simulink model "Task5_Subtask_1"  (R2023b)
settings: Solver=FixedStepDiscrete  StartTime=0.0  StopTime=(16+168+1)*24  RelTol=1e-3
settings Model: LastModifiedBy=AMEY THAKUR

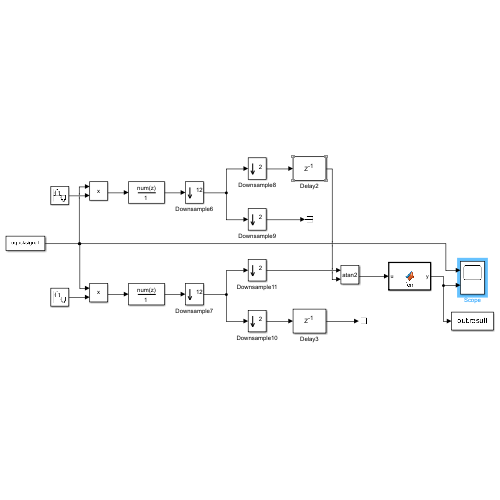
[thumbnail: Simulink's stored preview of the top-level diagram]
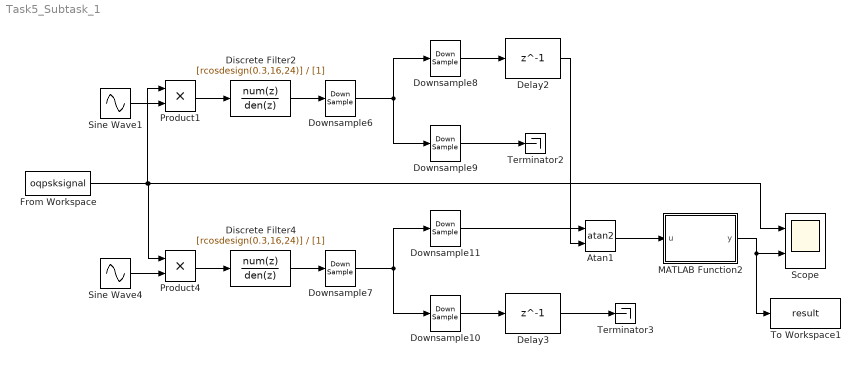
== system Task5_Subtask_1 ==
  Atan1 : Trigonometry  Operator=atan2
  Delay2 : Delay  DelayLength=1  UseCircularBuffer=on
  Delay3 : Delay  DelayLength=1  InitialCondition=0  UseCircularBuffer=on
  Discrete Filter2 : DiscreteFilter  Numerator=[rcosdesign(0.3,16,24)]  Denominator=[1]
  Discrete Filter4 : DiscreteFilter  Numerator=[rcosdesign(0.3,16,24)]  Denominator=[1]
  Downsample10 : DownSample  RateOptions=Allow multirate processing
  Downsample11 : DownSample  phase=1  RateOptions=Allow multirate processing
  Downsample6 : DownSample  N=12  RateOptions=Allow multirate processing
  Downsample7 : DownSample  N=12  RateOptions=Allow multirate processing
  Downsample8 : DownSample  RateOptions=Allow multirate processing
  Downsample9 : DownSample  phase=1  RateOptions=Allow multirate processing
  From Workspace : FromWorkspace  VariableName=oqpsksignal  SampleTime=1
  MATLAB Function2 : MATLAB Function  TreatAsAtomicUnit=on
  Product1 : Product
  Product4 : Product
  Scope : Scope  NumInputPorts=2
  Sine Wave1 : Sin  Amplitude=sqrt(2)  Frequency=2*pi*0.25  Phase=pi/2  SampleTime=1
  Sine Wave4 : Sin  Amplitude=-sqrt(2)  Frequency=2*pi*0.25  SampleTime=1
  Terminator2 : Terminator
  Terminator3 : Terminator
  To Workspace1 : ToWorkspace  VariableName=result  SampleTime=-1
      settings: Save2DSignal=2-D array (concatenate along first dimension)
  wires:
  Discrete Filter2/1 -> Downsample6/1
  Discrete Filter4/1 -> Downsample7/1
  Atan1/1 -> MATLAB Function2/1(u)
  Downsample10/1 -> Delay3/1
  Sine Wave4/1 -> Product4/2
  Product4/1 -> Discrete Filter4/1
  Downsample7/1 -> Downsample11/1, Downsample10/1
  Product1/1 -> Discrete Filter2/1
  Downsample9/1 -> Terminator2/1
  Downsample11/1 -> Atan1/1
  Delay3/1 -> Terminator3/1
  Sine Wave1/1 -> Product1/2
  MATLAB Function2/1(y) -> Scope/2, To Workspace1/1
  Downsample8/1 -> Delay2/1
  Downsample6/1 -> Downsample8/1, Downsample9/1
  Delay2/1 -> Atan1/2
  From Workspace/1 -> Scope/1, Product4/1, Product1/1

== matlab function Task5_Subtask_1/MATLAB Function2 ==
  data: u input; y output
function y = fcn(u)
y = zeros(size(u));
for i=1:length(u)
    if u(i)>= -pi/4 &&u(i)<pi/4
        y(i)=0;

    elseif u(i)>=(-pi/4) && u(i)<((3*pi)/4)
        y(i)=1;

    elseif u(i)>=((-3*pi)/4) && u(i)<(-pi/4)
        y(i)=2;
    else
        y(i)=3;
    end
end
